simulink model "TpLockInAmp"  (R2020b)
settings: Solver=ode4  StartTime=0.0  StopTime=inf  RelTol=1e-3
libraries: dspfdesign x2, dspsrcs4 x2
settings Model: Creator=LYX  LastModifiedBy=LYX
settings OptimizationCC: DefaultParameterBehavior=Inlined  EnhancedBackFolding=on  PassReuseOutputArgsAs=Individual arguments  ZeroExternalMemoryAtStartup=off  ZeroInternalMemoryAtStartup=off  OptimizeBlockOrder=speed  DifferentSizesBufferReuse=on  OptimizationCustomize=off  EfficientTunableParamExpr=on
settings DebuggingCC: ParameterTunabilityLossMsg=error
settings SFSimCC: MATLABDynamicMemAlloc=off
settings RTWCC: Description=Embedded Coder  SystemTargetFile=ert.tlc  GenCodeOnly=on  PackageGeneratedCodeAndArtifacts=on  TemplateMakefile=ert_default_tmf
settings CodeAppCC: ForceParamTrailComments=on  IgnoreCustomStorageClasses=off  OperatorAnnotations=on  SimulinkDataObjDesc=on  SFDataObjDesc=on  InsertBlockDesc=on
settings ERTTargetCC: TargetLangStandard=C99 (ISO)  GenerateSampleERTMain=on  InlinedParameterPlacement=NonHierarchical  ERTCustomFileTemplate=example_file_process.tlc

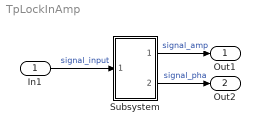
== system TpLockInAmp ==
  In1 : Inport
  Subsystem : Subsystem
  Out1 : Outport
  Out2 : Outport  Port=2
  wires:
  In1/1 -> Subsystem/1(In1)  "signal_input"
  Subsystem/1(Out1) -> Out1/1  "signal_amp"
  Subsystem/2(Out2) -> Out2/1  "signal_pha"

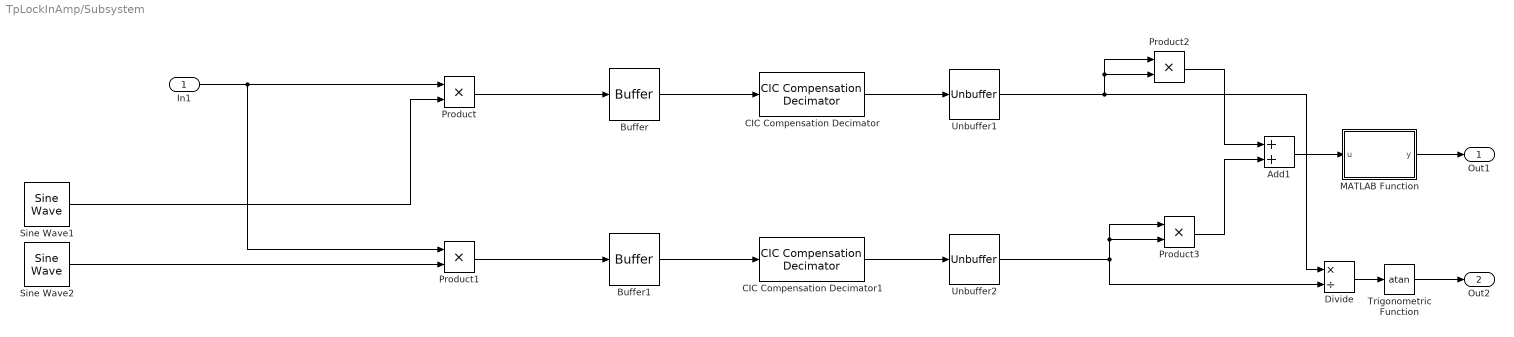
== system TpLockInAmp/Subsystem ==
  In1 : Inport
  Add1 : Sum
  Buffer : Buffer  N=8  OutputFrames=off
  Buffer1 : Buffer  N=8  OutputFrames=off
  CIC Compensation Decimator : dspfdesign/CIC Compensation Decimator  CICRateChangeFactor=4  CICNumSections=5  CICDifferentialDelay=1  DecimationFactor=4  DesignForMinimumOrder=on  FilterOrder=12  PassbandFrequency=1  StopbandFrequency=6  PassbandRipple=0.1  StopbandAttenuation=60  InheritSampleRate=on  SampleRate=1200000  SimulateUsing=Code generation  roundingMode=Floor  coeffsDataTypeStr=fixdt(1,16)
      settings: SourceProductBaseCode=DS
  CIC Compensation Decimator1 : dspfdesign/CIC Compensation Decimator  CICRateChangeFactor=4  CICNumSections=5  CICDifferentialDelay=1  DecimationFactor=4  DesignForMinimumOrder=on  FilterOrder=12  PassbandFrequency=1  StopbandFrequency=6  PassbandRipple=0.1  StopbandAttenuation=60  InheritSampleRate=on  SampleRate=1200000  SimulateUsing=Code generation  roundingMode=Floor  coeffsDataTypeStr=fixdt(1,16)
      settings: SourceProductBaseCode=DS
  Divide : Product  Inputs=*/
  MATLAB Function : MATLAB Function  TreatAsAtomicUnit=on
  Product{,1..3} (4 alike) : Product
  Sine Wave1 : dspsrcs4/Sine Wave  Amplitude=1  Frequency=20  Phase=0  SampleMode=Discrete  OutComplex=Real  CompMethod=Trigonometric fcn  TableSize=Speed  SampleTime=1/1000  SamplesPerFrame=1  ResetState=Restart at time zero  OutputFrames=off  dataType=double  wordLen=16  udDataType=sfix(16)  fracBitsMode=Best precision  numFracBits=15  OutDataTypeStr=double  LastOutDataTypeStr=double
  Sine Wave2 : dspsrcs4/Sine Wave  Amplitude=1  Frequency=20  Phase=pi/2  SampleMode=Discrete  OutComplex=Real  CompMethod=Trigonometric fcn  TableSize=Speed  SampleTime=1/1000  SamplesPerFrame=1  ResetState=Restart at time zero  OutputFrames=off  dataType=double  wordLen=16  udDataType=sfix(16)  fracBitsMode=Best precision  numFracBits=15  OutDataTypeStr=double  LastOutDataTypeStr=double
  Trigonometric Function : Trigonometry  Operator=atan
  Unbuffer1 : Unbuffer
  Unbuffer2 : Unbuffer
  Out1 : Outport
  Out2 : Outport  Port=2
  wires:
  Buffer1/1 -> CIC Compensation Decimator1/1
  Sine Wave1/1 -> Product/2
  Product/1 -> Buffer/1
  Unbuffer2/1 -> Divide/2, Product3/2, Product3/1
  MATLAB Function/1(y) -> Out1/1
  CIC Compensation Decimator/1 -> Unbuffer1/1
  Product1/1 -> Buffer1/1
  Add1/1 -> MATLAB Function/1(u)
  Buffer/1 -> CIC Compensation Decimator/1
  Unbuffer1/1 -> Divide/1, Product2/2, Product2/1
  Sine Wave2/1 -> Product1/2
  Product3/1 -> Add1/2
  Trigonometric Function/1 -> Out2/1
  Product2/1 -> Add1/1
  Divide/1 -> Trigonometric Function/1
  CIC Compensation Decimator1/1 -> Unbuffer2/1
  In1/1 -> Product1/1, Product/1

== matlab function TpLockInAmp/Subsystem/MATLAB Function ==
  data: u input; y output
function y = fcn(u)

y = 2 * sqrt(u);
